simulink model "trial_single_household"  (R2024b)
settings: Solver=VariableStepAuto  StartTime=0.0  StopTime=86400  RelTol=1e-3
libraries: spsVoltageMeasurementLib x2, spsThreePhaseSeriesRLCBranchLib x1, spsCurrentMeasurementLib x1, spsGroundLib x1, eePowerMeasurement x1, spsPVArrayLib x1, spsSeriesRLCLoadLib x1, spsThreePhaseDynamicLoadLib x1, spsThreePhaseSeriesRLCLoadLib x1, spsThreePhaseSourceLib x1, spspowerguiLib x1
settings Model: Creator=DELL  LastModifiedBy=DELL

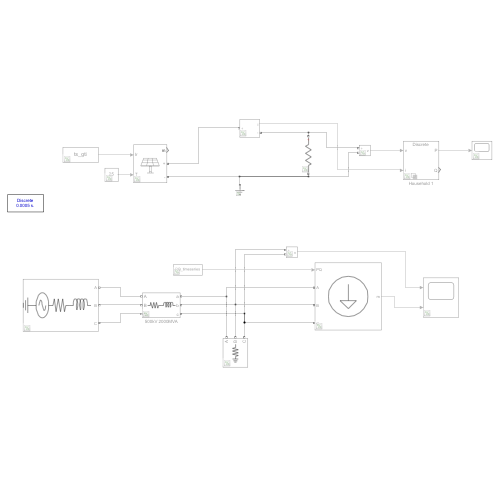
[thumbnail: Simulink's stored preview of the top-level diagram]
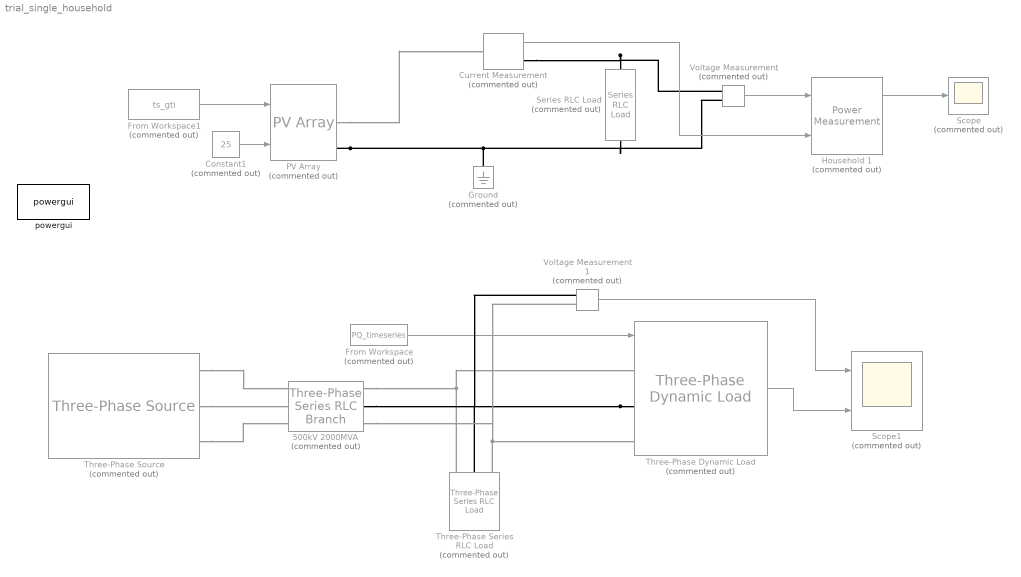
== system trial_single_household ==
  500kV 2000MVA : spsThreePhaseSeriesRLCBranchLib/Three-Phase Series RLC Branch  Commented=on  LConnTagsString=A|B|C  RConnTagsString=A|B|C  BranchType=RL  Resistance=500^2/2000/10  Inductance=500^2/2000/377  Capacitance=[]  Measurements=Branch voltages and currents
  Constant1 : Constant  Commented=on  Value=25
  Current Measurement : spsCurrentMeasurementLib/Current Measurement  Commented=on  PhasorSimulation=off  OutputType=Complex  PSBequivalent=0
  From Workspace : FromWorkspace  Commented=on  VariableName=PQ_timeseries  OutDataTypeStr=double
  From Workspace1 : FromWorkspace  Commented=on  VariableName=ts_gti  OutDataTypeStr=double
  Ground : spsGroundLib/Ground  Commented=on  LConnTagsString=a
  Household 1 : eePowerMeasurement/Power Measurement  Commented=on  LabelModeActiveChoice=Discrete  F=60  K=[0]  Ts=60
  PV Array : spsPVArrayLib/PV Array  Commented=on  Npar=2  Nser=6  PlotType=array @ 1000 W/m2 & specified temperatures  S_vec="[ 1000  500  100 ]"  Temp_C_vec="[ 45 25  ]"  ModuleName=SunPower SPR-415E-WHT-D  PlotWhenSelected=off  Pm=414.801  Ncell=128  Voc=85.3  Isc=6.09  Vm=72.9  Im=5.69  beta_Voc_pc=-0.229  alpha_Isc_pc=0.030706  beta_Voc=-0.19534  alpha_Isc=0.00187  IL=6.0978  I0=7.1698e-13  nI=0.87223  Rsh=419.7781  Rs=0.53711  RobustModel=off  RobustCellTemperature=313.3991  BAL=on  Tc=1e-6  Tfilter=5e-5
  Scope : Scope  Commented=on
  Scope1 : Scope  Commented=on  NumInputPorts=2
  Series RLC Load : spsSeriesRLCLoadLib/Series RLC Load  Commented=on  LConnTagsString=a  RConnTagsString=__new0  NominalVoltage=400  NominalFrequency=0.0000001  ActivePower=5000  InductivePower=0  CapacitivePower=0  Setx0=off  InitialVoltage=0  SetiL0=off  InitialCurrent=0  Measurements=Branch voltage and current  LoadType=constant I
  Three-Phase Dynamic Load : spsThreePhaseDynamicLoadLib/Three-Phase Dynamic Load  Commented=on  NominalVoltage=[ 500e3 60 ]  ActiveReactivePowers=[5e+007 2.5e+007]  PositiveSequence=[0.98441 -1.41063]  ExternalControl=on  NpNq=[1.3 2]  TimeConstants="[0  0  0  0]"  MinimumVoltage=0.7  Tfilter=1e-4  LoadFlowParameters=[4,0,0,0,0]
      settings: LibrarySourceBlock=|
      | sps_lib/Passives/Three-Phase
      | Dynamic Load
  Three-Phase Series RLC Load : spsThreePhaseSeriesRLCLoadLib/Three-Phase Series RLC Load  Commented=on  LConnTagsString=A|B|C  Configuration=Y (grounded)  NominalVoltage=400  Vabc=[1e3 1e3 1e3]  Vabcp=[1e3 1e3 1e3]  NominalFrequency=60  UnbalancedPower=off  ActivePower=1000  InductivePower=0  CapacitivePower=0  Pabc=[10e3 9e3 11e3]  QLabc=[100 90 110]  QCabc=[100 90 110]  Pabcp=[10e3 9e3 11e3]  QLabcp=[100 90 110]  QCabcp=[100 90 110]  Measurements=None  LoadType=constant Z
  Three-Phase Source : spsThreePhaseSourceLib/Three-Phase Source  Commented=on  InternalConnection=Yg  VoltagePhases=off  Voltage=400  PhaseAngle=0  Voltage_phases=[25e3 25e3 25e3]/sqrt(3)  PhaseAngles_phases=[0 -120 +120]  Frequency=60  NonIdealSource=on  SpecifyImpedance=off  Resistance=0.8929  Inductance=16.58e-3  ShortCircuitLevel=100e6  BaseVoltage=25e3  XRratio=7  BusType=PV  Pref=10e3  Qref=0  Prefabc=[10e3, 10e3, 10e3]  Qrefabc=[0, 0, 0]  Qmin=-inf  Qmax=inf
  Voltage Measurement : spsVoltageMeasurementLib/Voltage Measurement  Commented=on  PhasorSimulation=off  OutputType=Complex  PSBequivalent=0
  Voltage Measurement1 : spsVoltageMeasurementLib/Voltage Measurement  Commented=on  PhasorSimulation=off  OutputType=Complex  PSBequivalent=0
  powergui : spspowerguiLib/powergui  Priority=1  SimulationMode=Discrete  SampleTime=5e-4  frequency=60  Iterations=50  frequencyindice=60  Pbase=100e6  ErrMax=1e-4  UnitsV=kV  UnitsW=MW  buscounter=0  FunctionMessages=off  echomessages=off  EnableUseOfTLC=off  CurrentSourceSwitches=off  DisableSnubberDevices=off  DisableRonSwitches=off  DisableVfSwitches=off  DisplayEquations=off  AutomaticDiscreteSolvers=off  SolverType=Tustin/Backward Euler (TBE)  Interpol=off  ExternalGateDelay=off  methode=off  Ts=100  x0status=blocks  SPID=on  SwTol=0  HookPort=off  NonlinearTolerance=1e-4  nMaxIteration=100  ContinueOnMaxIteration=off  RestoreLinks=warning  ResistiveCurrentMeasurement=off  Frange=[0:2:500]  Ylog=off  Xlog=on  ShowGrid=off  save=off  variable=ZData  structure=0  ZoomFFT=off  StartTime=0.0  cycles=1  DisplayStyle=1  fundamental=60  FreqAxis=off  MaxFrequency=1000  frequencyindicesteady=1  RmsSteady=1  display=off
  wires:
  Household 1/1 -> Scope/1
  Constant1/1 -> PV Array/2
  Voltage Measurement/1 -> Household 1/1
  Current Measurement/1 -> Household 1/2
  From Workspace1/1 -> PV Array/1
  From Workspace/1 -> Three-Phase Dynamic Load/1
  Three-Phase Dynamic Load/1 -> Scope1/2
  Voltage Measurement1/1 -> Scope1/1
  connections:
  PV Array/RConn2 -- Series RLC Load/RConn1 -- Voltage Measurement/LConn2 -- Ground/LConn1
  Series RLC Load/LConn1 -- Current Measurement/RConn1 -- Voltage Measurement/LConn1
  PV Array/RConn1 -- Current Measurement/LConn1
  Three-Phase Series RLC Load/LConn1 -- Three-Phase Dynamic Load/LConn1 -- 500kV 2000MVA/RConn1
  Three-Phase Dynamic Load/LConn2 -- 500kV 2000MVA/RConn2 -- Voltage Measurement1/LConn1 -- Three-Phase Series RLC Load/LConn2
  Three-Phase Series RLC Load/LConn3 -- 500kV 2000MVA/RConn3 -- Voltage Measurement1/LConn2 -- Three-Phase Dynamic Load/LConn3
  Three-Phase Source/RConn1 -- 500kV 2000MVA/LConn1
  Three-Phase Source/RConn2 -- 500kV 2000MVA/LConn2
  Three-Phase Source/RConn3 -- 500kV 2000MVA/LConn3
